simulink model "RealModel"  (R2019a)
settings: Solver=ode45  StartTime=0.0  StopTime=50  FixedStep=5e-5  MaxStep=1e-4  MinStep=1e-6  RelTol=1e-10
InitFcn:
  | Rs = 0.011
  | Ld = 0.018
  | Lq = 0.018
  | Fi = 0.055
  | p = 4
  | J = 0.102
  | b = 0.18
  | 
  | tC = 20
  | k3 = -1.586440829524976
  | k4 = -0.541242258944882
  | k5 = -0.541242258944882
  | k6 = -0.328094464592671
  | 
  | ide = 2.930555555555555
  | iqe = 0.605243293597248
settings Model: Creator=LiLid  LastModifiedBy=LiLid

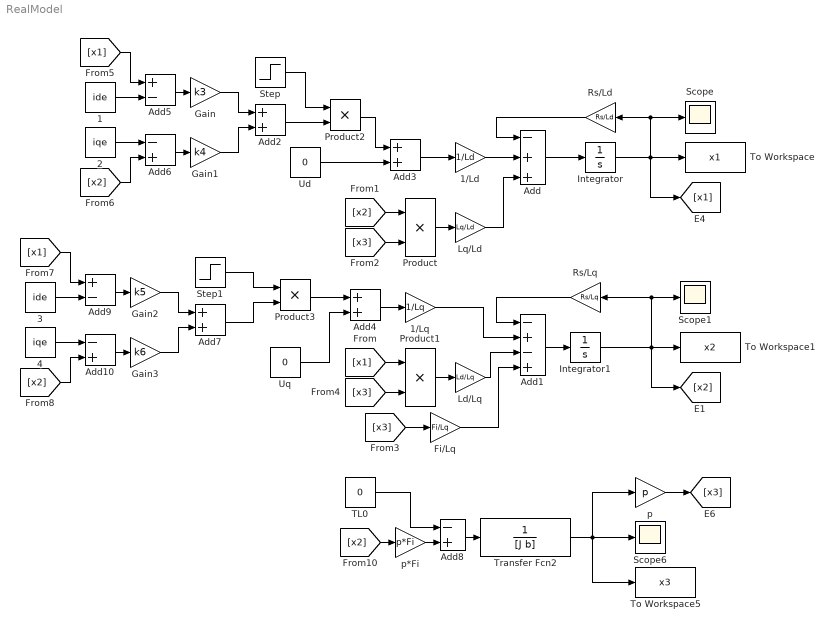
== system RealModel ==
  1 : Constant  Value=ide
  1/Ld : Gain  Gain=1/Ld
  1/Lq : Gain  Gain=1/Lq
  2 : Constant  Value=iqe
  3 : Constant  Value=ide
  4 : Constant  Value=iqe
  Add : Sum  Inputs=-++
  Add1 : Sum  Inputs=-+-+
  Add10 : Sum  Inputs=-+
  Add{2..4,7} (4 alike) : Sum
  Add5 : Sum  Inputs=+-
  Add6 : Sum  Inputs=-+
  Add8 : Sum  Inputs=-+
  Add9 : Sum  Inputs=+-
  Fi/Lq : Gain  Gain=Fi/Lq
  Gain : Gain  Gain=k3
  Gain1 : Gain  Gain=k4
  Gain2 : Gain  Gain=k5
  Gain3 : Gain  Gain=k6
  Integrator : Integrator  InitialCondition=0.15
  Integrator1 : Integrator  InitialCondition=0.14
  Ld/Lq : Gain  Gain=Ld/Lq
  Lq/Ld : Gain  Gain=Lq/Ld
  Product{,1..3} (4 alike) : Product
  Rs/Ld : Gain  Gain=Rs/Ld
  Rs/Lq : Gain  Gain=Rs/Lq
  Scope : Scope
  Scope1 : Scope
  Scope6 : Scope
  Step : Step  Time=tC  SampleTime=0
  Step1 : Step  Time=tC  SampleTime=0
  TL0 : Constant  Value=0
  To Workspace : ToWorkspace  VariableName=x1  SampleTime=-1
      settings: Save2DSignal=2-D array (concatenate along first dimension)
  To Workspace1 : ToWorkspace  VariableName=x2  SampleTime=-1
      settings: Save2DSignal=2-D array (concatenate along first dimension)
  To Workspace5 : ToWorkspace  VariableName=x3  SampleTime=-1
      settings: Save2DSignal=2-D array (concatenate along first dimension)
  Transfer Fcn2 : TransferFcn  Denominator=[J b]
  Ud : Constant  Value=0
  Uq : Constant  Value=0
  p : Gain  Gain=p
  p*Fi : Gain  Gain=p*Fi
  wires:
  Integrator/1 -> To Workspace/1, [x1], Scope/1, Rs/Ld/1
  Add/1 -> Integrator/1
  Rs/Ld/1 -> Add/1
  Product/1 -> Lq/Ld/1
  [x2] -> Product/1
  [x3] -> Product/2
  Integrator1/1 -> To Workspace1/1, Rs/Lq/1, Scope1/1, [x2]
  Rs/Lq/1 -> Add1/1
  Add1/1 -> Integrator1/1
  [x1] -> Product1/1
  [x3] -> Product1/2
  [x3] -> Fi/Lq/1
  Fi/Lq/1 -> Add1/4
  Lq/Ld/1 -> Add/3
  1/Ld/1 -> Add/2
  1/Lq/1 -> Add1/2
  Product1/1 -> Ld/Lq/1
  Ld/Lq/1 -> Add1/3
  p/1 -> [x3]
  p*Fi/1 -> Add8/2
  [x2] -> p*Fi/1
  Add8/1 -> Transfer Fcn2/1
  Transfer Fcn2/1 -> Scope6/1, p/1, To Workspace5/1
  TL0/1 -> Add8/1
  Gain1/1 -> Add2/2
  Gain/1 -> Add2/1
  Add2/1 -> Product2/2
  Ud/1 -> Add3/2
  Add3/1 -> 1/Ld/1
  Step/1 -> Product2/1
  Product2/1 -> Add3/1
  Add4/1 -> 1/Lq/1
  Uq/1 -> Add4/2
  Product3/1 -> Add4/1
  Add5/1 -> Gain/1
  [x1] -> Add5/1
  1/1 -> Add5/2
  Add6/1 -> Gain1/1
  2/1 -> Add6/1
  [x2] -> Add6/2
  3/1 -> Add9/2
  [x2] -> Add10/2
  4/1 -> Add10/1
  Gain2/1 -> Add7/1
  Add10/1 -> Gain3/1
  [x1] -> Add9/1
  Add9/1 -> Gain2/1
  Gain3/1 -> Add7/2
  Add7/1 -> Product3/2
  Step1/1 -> Product3/1
